simulink model "simple_time_delay_model"  (R2023b)
settings: Solver=VariableStepAuto  StartTime=0.0  StopTime=10.0  RelTol=1e-3
undefined symbols (not defined in the file): Adtilde, Bdtildey, Cdtilde, Ddtilde, Dm, ei, M, nutildei, Pm, td, xi
libraries: simulink x1
settings Model: Creator=tamas  LastModifiedBy=tamas

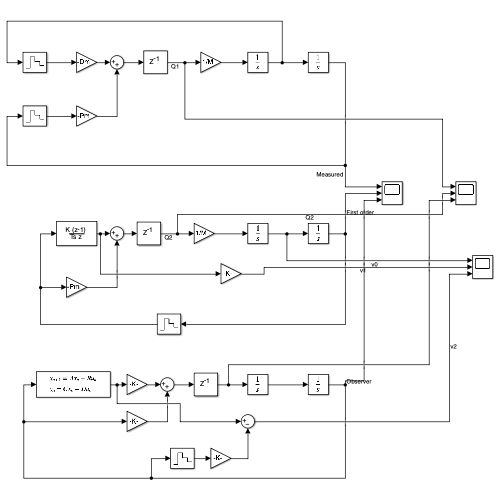
[thumbnail: Simulink's stored preview of the top-level diagram]
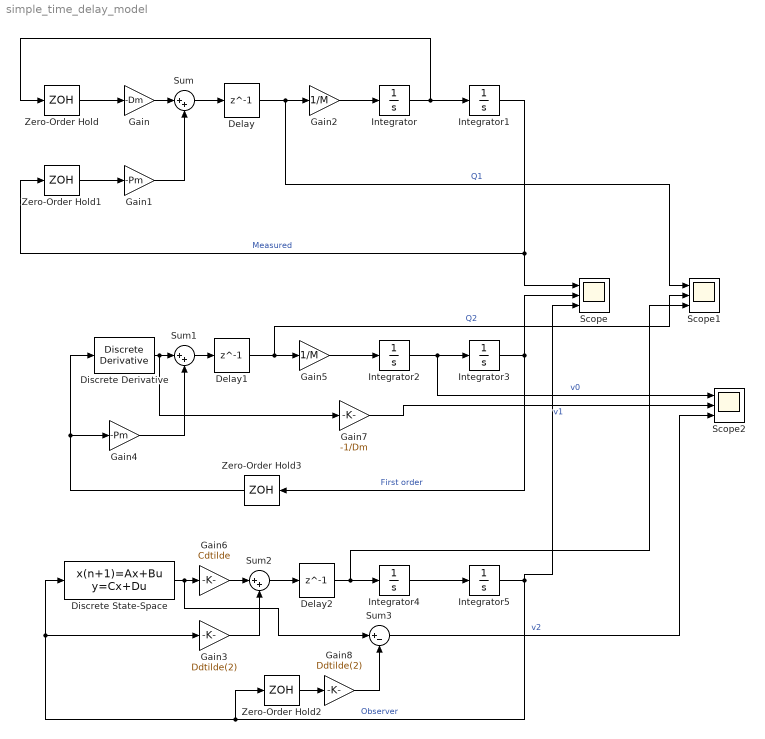
== system simple_time_delay_model ==
  Delay : Delay  DelayLength=1  InitialCondition=0  SampleTime=td
  Delay1 : Delay  DelayLength=1  InitialCondition=0  SampleTime=td
  Delay2 : Delay  DelayLength=1  InitialCondition=0  SampleTime=td
  Discrete Derivative : simulink/Discrete/Discrete Derivative  gainval=-Dm  ICPrevScaledInput=ei - xi(1)  OutMin=[]  OutMax=[]  OutDataType=fixdt(1, 16)  OutScaling=2^-10  DoSatur=off
  Discrete State-Space : DiscreteStateSpace  A=Adtilde  B=Bdtildey  D=0  InitialCondition=nutildei  SampleTime=td
  Gain : Gain  Gain=-Dm
  Gain1 : Gain  Gain=-Pm
  Gain2 : Gain  Gain=1/M
  Gain3 : Gain  Gain=Ddtilde(2)
  Gain4 : Gain  Gain=-Pm
  Gain5 : Gain  Gain=1/M
  Gain6 : Gain  Gain=Cdtilde
  Gain7 : Gain  Gain=-1/Dm
  Gain8 : Gain  Gain=Ddtilde(2)
  Integrator : Integrator  InitialCondition=xi(2)
  Integrator1 : Integrator  InitialCondition=xi(1)
  Integrator2 : Integrator  InitialCondition=xi(2)
  Integrator3 : Integrator  InitialCondition=xi(1)
  Integrator4 : Integrator  InitialCondition=xi(2)
  Integrator5 : Integrator  InitialCondition=xi(1)
  Scope : Scope  NumInputPorts=3
  Scope1 : Scope  NumInputPorts=3
  Scope2 : Scope  NumInputPorts=3
  Sum : Sum  Inputs=|++
  Sum1 : Sum  Inputs=|++
  Sum2 : Sum  Inputs=|++
  Sum3 : Sum  Inputs=|+-
  Zero-Order Hold{,1..3} (4 alike) : ZeroOrderHold  SampleTime=td
  wires:
  Integrator1/1 -> Zero-Order Hold1/1, Scope/1  "Measured"
  Zero-Order Hold1/1 -> Gain1/1
  Gain1/1 -> Sum/2
  Gain/1 -> Sum/1
  Zero-Order Hold/1 -> Gain/1
  Integrator/1 -> Integrator1/1, Zero-Order Hold/1
  Delay/1 -> Scope1/1, Gain2/1  "Q1"
  Sum/1 -> Delay/1
  Integrator3/1 -> Zero-Order Hold3/1, Scope/2  "First order"
  Gain4/1 -> Sum1/2
  Integrator2/1 -> Scope2/1, Integrator3/1  "v0"
  Zero-Order Hold3/1 -> Gain4/1, Discrete Derivative/1
  Sum1/1 -> Delay1/1
  Delay1/1 -> Scope1/2, Gain5/1  "Q2"
  Delay2/1 -> Scope1/3, Integrator4/1
  Integrator5/1 -> Scope/3, Zero-Order Hold2/1, Gain3/1, Discrete State-Space/1  "Observer"
  Discrete State-Space/1 -> Sum3/1, Gain6/1
  Integrator4/1 -> Integrator5/1
  Gain2/1 -> Integrator/1
  Gain5/1 -> Integrator2/1
  Gain6/1 -> Sum2/1
  Sum2/1 -> Delay2/1
  Gain3/1 -> Sum2/2
  Discrete Derivative/1 -> Gain7/1, Sum1/1
  Gain7/1 -> Scope2/2  "v1"
  Gain8/1 -> Sum3/2
  Zero-Order Hold2/1 -> Gain8/1
  Sum3/1 -> Scope2/3  "v2"
